simulink model "integrated"  (R2020b)
settings: Solver=VariableStepAuto  StartTime=0.0  StopTime=100  RelTol=1e-3
undefined symbols (not defined in the file or in its folder): sigbuilder_block
settings Model: EnablePacing=on  PacingRate=2  Creator=99003729  LastModifiedBy=99003729

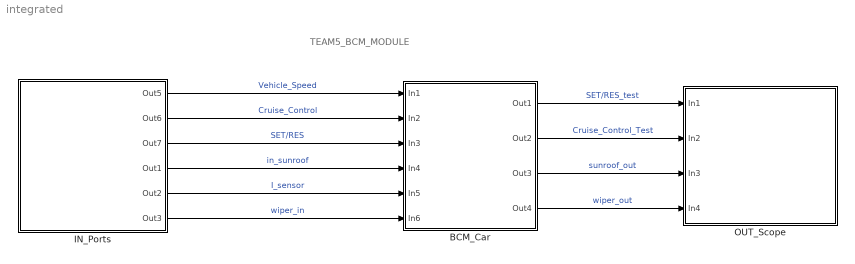
== system integrated ==
  note: TEAM5_BCM_MODULE
  BCM_Car : Subsystem
  IN_Ports : Subsystem
  OUT_Scope : Subsystem
  wires:
  IN_Ports/1(Out5) -> BCM_Car/1(In1)  "Vehicle_Speed"
  IN_Ports/3(Out7) -> BCM_Car/3(In3)  "SET/RES"
  IN_Ports/2(Out6) -> BCM_Car/2(In2)  "Cruise_Control"
  BCM_Car/1(Out1) -> OUT_Scope/1(In1)  "SET/RES_test"
  BCM_Car/2(Out2) -> OUT_Scope/2(In2)  "Cruise_Control_Test"
  IN_Ports/4(Out1) -> BCM_Car/4(In4)  "in_sunroof"
  IN_Ports/5(Out2) -> BCM_Car/5(In5)  "I_sensor"
  IN_Ports/6(Out3) -> BCM_Car/6(In6)  "wiper_in"
  BCM_Car/3(Out3) -> OUT_Scope/3(In3)  "sunroof_out"
  BCM_Car/4(Out4) -> OUT_Scope/4(In4)  "wiper_out"

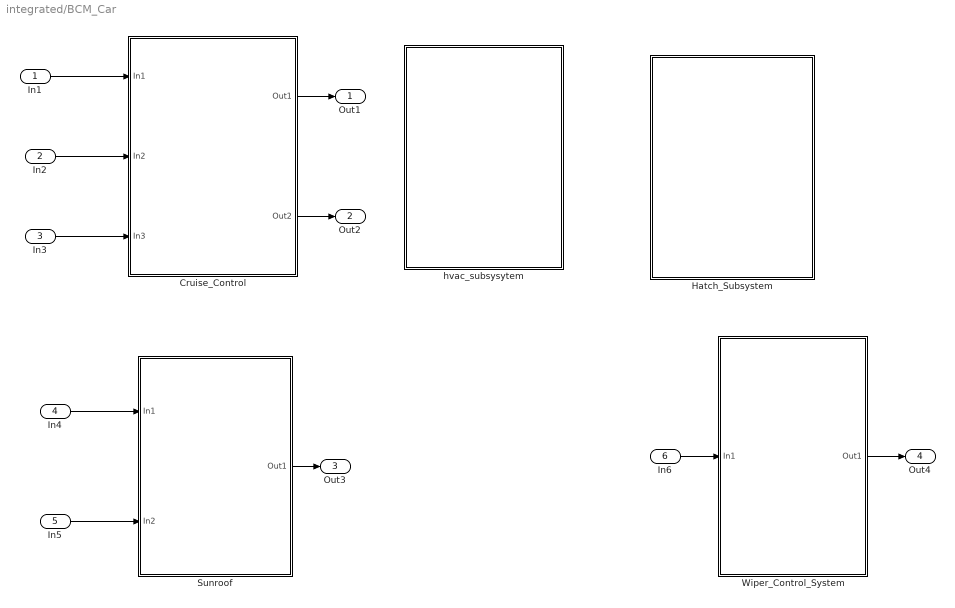
== system integrated/BCM_Car ==
  In1 : Inport
  In2 : Inport  Port=2
  In3 : Inport  Port=3
  In4 : Inport  Port=4
  In5 : Inport  Port=5
  In6 : Inport  Port=6
  Cruise_Control : Subsystem
  Hatch_Subsystem : Subsystem
  Sunroof : Subsystem
  Wiper_Control_System : Subsystem
  hvac_subsysytem : Subsystem
  Out1 : Outport
  Out2 : Outport  Port=2
  Out3 : Outport  Port=3
  Out4 : Outport  Port=4
  wires:
  In1/1 -> Cruise_Control/1(In1)
  In2/1 -> Cruise_Control/2(In2)
  In3/1 -> Cruise_Control/3(In3)
  Cruise_Control/1(Out1) -> Out1/1
  Cruise_Control/2(Out2) -> Out2/1
  In4/1 -> Sunroof/1(In1)
  In5/1 -> Sunroof/2(In2)
  Sunroof/1(Out1) -> Out3/1
  In6/1 -> Wiper_Control_System/1(In1)
  Wiper_Control_System/1(Out1) -> Out4/1

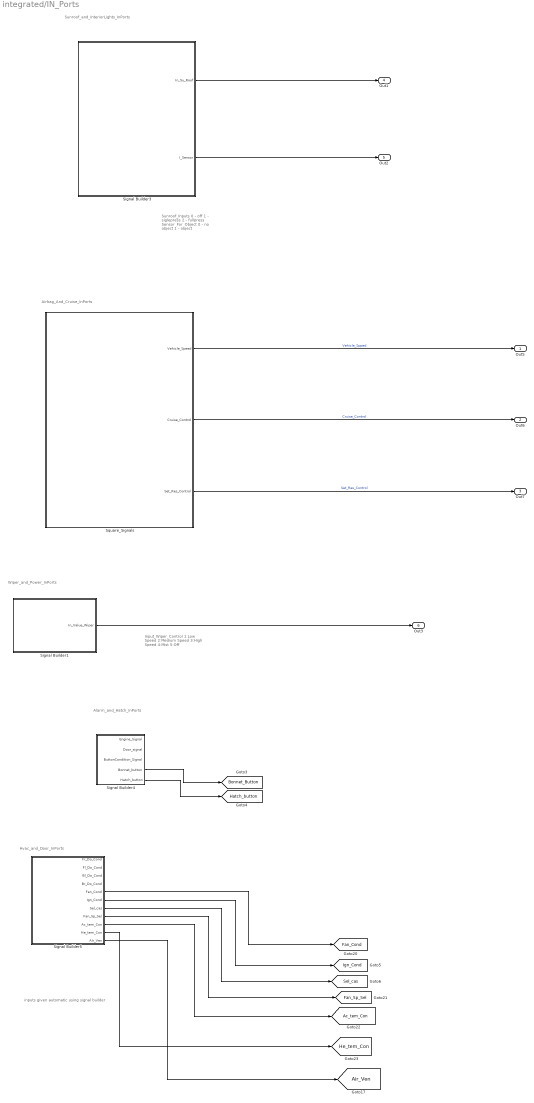
== system integrated/IN_Ports ==
  note: Hvac_and_Door_InPorts
  note: Alarm_and_Hatch_InPorts
  note: Sunroof_and_InteriorLights_InPorts
  note: Wiper_and_Power_InPorts
  note: Airbag_And_Cruise_InPorts
  note: Input_Wiper_Control
      | 1:Low Speed
      | 2:Medium Speed
      | 3:High Speed
      | 4:Mist
      | 5:Off
  note: Sunroof_Inputs
      | 0 - off
      | 1 - siglepress
      | 2 - fullpress
      | Sensor_For_Object
      | 0 - no object
      | 1 - object
  note: inputs given automatic using signal builder
  Signal Builder1 : Subsystem  Tag=STV Subsys  LoadFcn=sigbuilder_block('load');  StartFcn=sigbuilder_block('start');  StopFcn=sigbuilder_block('stop');  ClipboardFcn=sigbuilder_block('clipboard');  mask(Sigbuilder block){tuvar=[0:10]}
      mask help: Simulink:masks:SigbuilderBlock_MD
      mask init:
      | if ~strcmp(get_param(bdroot(gcbh),'SimulationStatus'),'stopped') tuvar = sigbuilder_block('maskInit'); end
      settings: CopyFcn=sigbuilder_block('copy');  DeleteFcn=sigbuilder_block('delete');  ModelCloseFcn=sigbuilder_block('modelClose');  PreSaveFcn=sigbuilder_block('preSave');  PauseFcn=sigbuilder_block('pause');  ContinueFcn=sigbuilder_block('continue');  NameChangeFcn=sigbuilder_block('namechange');  OpenFcn=sigbuilder_block('open',[0.75 30.75 718.5 715.5 ]);  CloseFcn=sigbuilder_block('close');
      mask Display: plot(0, 0, 100, 100,[2, 2, 32, 32, 2], [68, 8, 8, 68, 68],[32, 2], [38, 38], [32, 19, 2],[53, 60, 44], [32, 17, 17, 2],[16, 16, 31, 31]);txt = getActiveGroup(gcbh);text(2, 100, txt,'verticalAlignment', 'top');
  Signal Builder3 : Subsystem  Tag=STV Subsys  LoadFcn=sigbuilder_block('load');  StartFcn=sigbuilder_block('start');  StopFcn=sigbuilder_block('stop');  ClipboardFcn=sigbuilder_block('clipboard');  mask(Sigbuilder block){tuvar=[0:10]}
      mask help: Simulink:masks:SigbuilderBlock_MD
      mask init:
      | if ~strcmp(get_param(bdroot(gcbh),'SimulationStatus'),'stopped') tuvar = sigbuilder_block('maskInit'); end
      settings: CopyFcn=sigbuilder_block('copy');  DeleteFcn=sigbuilder_block('delete');  ModelCloseFcn=sigbuilder_block('modelClose');  PreSaveFcn=sigbuilder_block('preSave');  PauseFcn=sigbuilder_block('pause');  ContinueFcn=sigbuilder_block('continue');  NameChangeFcn=sigbuilder_block('namechange');  OpenFcn=sigbuilder_block('open',[591 352.5 550.5 359.25 ]);  CloseFcn=sigbuilder_block('close');
      mask Display: plot(0, 0, 100, 100,[2, 2, 32, 32, 2], [68, 8, 8, 68, 68],[32, 2], [38, 38], [32, 19, 2],[53, 60, 44], [32, 17, 17, 2],[16, 16, 31, 31]);txt = getActiveGroup(gcbh);text(2, 100, txt,'verticalAlignment', 'top');
  Signal Builder4 : Subsystem  Tag=STV Subsys  LoadFcn=sigbuilder_block('load');  StartFcn=sigbuilder_block('start');  StopFcn=sigbuilder_block('stop');  ClipboardFcn=sigbuilder_block('clipboard');  mask(Sigbuilder block){tuvar=[0:10]}
      mask help: Simulink:masks:SigbuilderBlock_MD
      mask init:
      | if ~strcmp(get_param(bdroot(gcbh),'SimulationStatus'),'stopped') tuvar = sigbuilder_block('maskInit'); end
      settings: CopyFcn=sigbuilder_block('copy');  DeleteFcn=sigbuilder_block('delete');  ModelCloseFcn=sigbuilder_block('modelClose');  PreSaveFcn=sigbuilder_block('preSave');  PauseFcn=sigbuilder_block('pause');  ContinueFcn=sigbuilder_block('continue');  NameChangeFcn=sigbuilder_block('namechange');  OpenFcn=sigbuilder_block('open',[437.6 199.2 550.4 400 ]);  CloseFcn=sigbuilder_block('close');
      mask Display: plot(0, 0, 100, 100,[2, 2, 32, 32, 2], [68, 8, 8, 68, 68],[32, 2], [38, 38], [32, 19, 2],[53, 60, 44], [32, 17, 17, 2],[16, 16, 31, 31]);txt = getActiveGroup(gcbh);text(2, 100, txt,'verticalAlignment', 'top');
  Signal Builder5 : Subsystem  Tag=STV Subsys  LoadFcn=sigbuilder_block('load');  StartFcn=sigbuilder_block('start');  StopFcn=sigbuilder_block('stop');  ClipboardFcn=sigbuilder_block('clipboard');  mask(Sigbuilder block){tuvar=[0:10]}
      mask help: Simulink:masks:SigbuilderBlock_MD
      mask init:
      | if ~strcmp(get_param(bdroot(gcbh),'SimulationStatus'),'stopped') tuvar = sigbuilder_block('maskInit'); end
      settings: CopyFcn=sigbuilder_block('copy');  DeleteFcn=sigbuilder_block('delete');  ModelCloseFcn=sigbuilder_block('modelClose');  PreSaveFcn=sigbuilder_block('preSave');  PauseFcn=sigbuilder_block('pause');  ContinueFcn=sigbuilder_block('continue');  NameChangeFcn=sigbuilder_block('namechange');  OpenFcn=sigbuilder_block('open',[544.5 115.5 550.5 399.75 ]);  CloseFcn=sigbuilder_block('close');
      mask Display: plot(0, 0, 100, 100,[2, 2, 32, 32, 2], [68, 8, 8, 68, 68],[32, 2], [38, 38], [32, 19, 2],[53, 60, 44], [32, 17, 17, 2],[16, 16, 31, 31]);txt = getActiveGroup(gcbh);text(2, 100, txt,'verticalAlignment', 'top');
  Square_Signals : Subsystem  Tag=STV Subsys  LoadFcn=sigbuilder_block('load');  StartFcn=sigbuilder_block('start');  StopFcn=sigbuilder_block('stop');  ClipboardFcn=sigbuilder_block('clipboard');  mask(Sigbuilder block){tuvar=[0:10]}
      mask help: Simulink:masks:SigbuilderBlock_MD
      mask init:
      | if ~strcmp(get_param(bdroot(gcbh),'SimulationStatus'),'stopped') tuvar = sigbuilder_block('maskInit'); end
      settings: CopyFcn=sigbuilder_block('copy');  DeleteFcn=sigbuilder_block('delete');  ModelCloseFcn=sigbuilder_block('modelClose');  PreSaveFcn=sigbuilder_block('preSave');  PauseFcn=sigbuilder_block('pause');  ContinueFcn=sigbuilder_block('continue');  NameChangeFcn=sigbuilder_block('namechange');  OpenFcn=sigbuilder_block('open',[6 30 1012.5 447.75 ]);  CloseFcn=sigbuilder_block('close');
      mask Display: plot(0, 0, 100, 100,[2, 2, 32, 32, 2], [68, 8, 8, 68, 68],[32, 2], [38, 38], [32, 19, 2],[53, 60, 44], [32, 17, 17, 2],[16, 16, 31, 31]);txt = getActiveGroup(gcbh);text(2, 100, txt,'verticalAlignment', 'top');
  Out5 : Outport
  Out6 : Outport  Port=2
  Out7 : Outport  Port=3
  Out1 : Outport  Port=4
  Out2 : Outport  Port=5
  Out3 : Outport  Port=6
  tag scope: Ac_tem_Con=global, Air_Ven=global, Bonnet_Button=global, Fan_Cond=global, Fan_Sp_Sel=global, Hatch_button=global, He_tem_Con=global, Ign_Cond=global, Sel_cas=global
  wires:
  Square_Signals/2(Cruise_Control) -> Out6/1  "Cruise_Control"
  Square_Signals/1(Vehicle_Speed) -> Out5/1  "Vehicle_Spped"
  Square_Signals/3(Set_Res_Control) -> Out7/1  "Set_Res_Control"
  Signal Builder1/1(In_Value_Wiper) -> Out3/1
  Signal Builder3/1(In_Su_Roof) -> Out1/1
  Signal Builder3/2(I_Sensor) -> Out2/1
  Signal Builder4/4(Bonnet_button) -> [Bonnet_Button]
  Signal Builder4/5(Hatch_button) -> [Hatch_button]
  Signal Builder5/10(He_tem_Con) -> [He_tem_Con]
  Signal Builder5/11(AIr_Ven) -> [Air_Ven]
  Signal Builder5/9(Ac_tem_Con) -> [Ac_tem_Con]
  Signal Builder5/5(Fan_Cond) -> [Fan_Cond]
  Signal Builder5/8(Fan_Sp_Sel) -> [Fan_Sp_Sel]
  Signal Builder5/7(Sel_cas) -> [Sel_cas]
  Signal Builder5/6(Ign_Cond) -> [Ign_Cond]

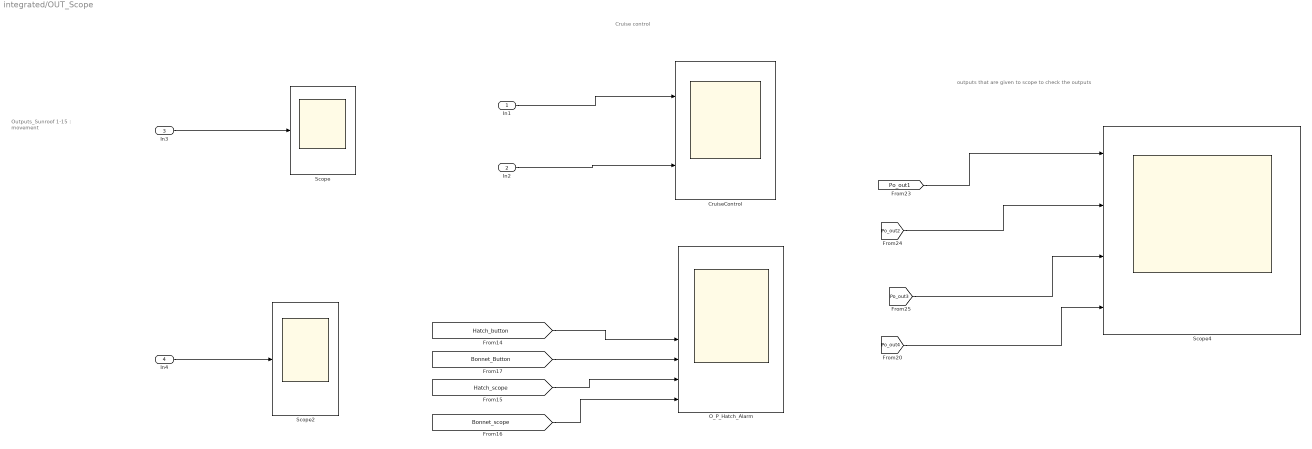
== system integrated/OUT_Scope ==
  note: Cruise control
  note: Outputs_Sunroof
      | 1-15 : movement
  note: outputs that are given to scope to check the outputs
  In1 : Inport
  In2 : Inport  Port=2
  In3 : Inport  Port=3
  In4 : Inport  Port=4
  CruiseControl : Scope  NumInputPorts=2
  O_P_Hatch_Alarm : Scope  NumInputPorts=8
  Scope : Scope
  Scope2 : Scope
  Scope4 : Scope  NumInputPorts=4
  wires:
  In4/1 -> Scope2/1
  In3/1 -> Scope/1
  [Bonnet_Button] -> O_P_Hatch_Alarm/6
  [Bonnet_scope] -> O_P_Hatch_Alarm/8
  [Hatch_button] -> O_P_Hatch_Alarm/5
  [Hatch_scope] -> O_P_Hatch_Alarm/7
  [Po_out3] -> Scope4/3
  [Po_out4] -> Scope4/4
  [Po_out1] -> Scope4/1
  [Po_out2] -> Scope4/2
  In1/1 -> CruiseControl/1
  In2/1 -> CruiseControl/2

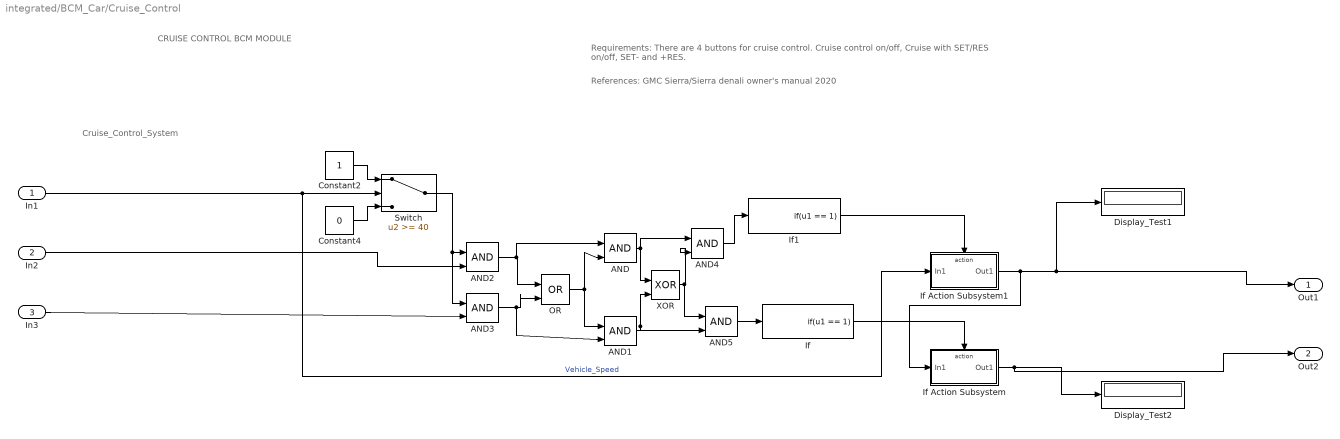
== system integrated/BCM_Car/Cruise_Control ==
  note: Cruise_Control_System
  note: CRUISE CONTROL BCM MODULE
  note: References: GMC Sierra/Sierra denali owner's manual 2020
  note: Requirements: There are 4 buttons for cruise control. Cruise control on/off, Cruise with SET/RES on/off, SET- and +RES.
  In1 : Inport
  In2 : Inport  Port=2
  In3 : Inport  Port=3
  AND{,1..5} (6 alike) : Logic  IconShape=distinctive  AllPortsSameDT=off  OutDataTypeStr=boolean
  Constant2 : Constant
  Constant4 : Constant  Value=0
  Display_Test1 : Display
  Display_Test2 : Display
  If : If  IfExpression=u1 == 1  ShowElse=off
  If Action Subsystem : Subsystem  TreatAsAtomicUnit=on
  If Action Subsystem1 : Subsystem  TreatAsAtomicUnit=on
  If1 : If  IfExpression=u1 == 1  ShowElse=off
  OR : Logic  Operator=OR  IconShape=distinctive  AllPortsSameDT=off  OutDataTypeStr=boolean
  Switch : Switch  Threshold=40
  XOR : Logic  Operator=XOR  IconShape=distinctive  AllPortsSameDT=off  OutDataTypeStr=boolean
  Out1 : Outport
  Out2 : Outport  Port=2
  wires:
  In3/1 -> AND3/2
  AND5/1 -> If/1
  If1/1 -> If Action Subsystem1/Action
  If/1 -> If Action Subsystem/Action
  If Action Subsystem/1(Out1) -> Out2/1, Display_Test2/1
  AND/1 -> AND4/1, XOR/1
  XOR/1 -> AND5/1, AND4/2
  In1/1 -> If Action Subsystem1/1(In1), Switch/2  "Vehicle_Speed"
  OR/1 -> AND1/1, AND/2
  AND2/1 -> AND/1, OR/1
  In2/1 -> AND2/2
  Constant4/1 -> Switch/3
  AND3/1 -> AND1/2, OR/2
  AND1/1 -> XOR/2, AND5/2
  Switch/1 -> AND3/1, AND2/1
  Constant2/1 -> Switch/1
  AND4/1 -> If1/1
  If Action Subsystem1/1(Out1) -> If Action Subsystem/1(In1), Out1/1, Display_Test1/1

== system integrated/BCM_Car/Hatch_Subsystem ==
  H_B_condition : Stateflow chart  TreatAsAtomicUnit=on
  Hatch_Bonnet_condition : Display
  OR : Logic  Operator=OR  IconShape=distinctive  AllPortsSameDT=off  OutDataTypeStr=boolean
  tag scope: Bonnet_scope=global, Hatch_scope=global
  wires:
  [Bonnet_Button] -> H_B_condition/1(BonnetButton)
  OR/1 -> Hatch_Bonnet_condition/1
  H_B_condition/1(y) -> [Bonnet_scope], OR/1
  H_B_condition/2(x) -> [Hatch_scope], OR/2
  [Hatch_button] -> H_B_condition/2(hatchButton)

== system integrated/BCM_Car/Sunroof ==
  In1 : Inport
  In2 : Inport  Port=2
  Function_Sun : MATLAB Function  TreatAsAtomicUnit=on
  Out1 : Outport
  wires:
  Function_Sun/1(y) -> Out1/1  "Out_Sun"
  In2/1 -> Function_Sun/2(v)
  In1/1 -> Function_Sun/1(u)

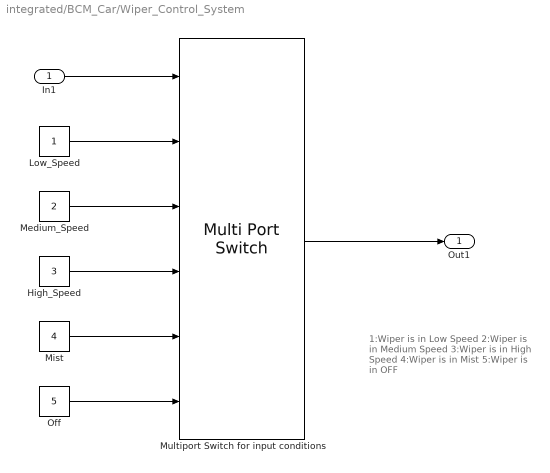
== system integrated/BCM_Car/Wiper_Control_System ==
  note: 1:Wiper is in Low Speed
      | 2:Wiper is in Medium Speed
      | 3:Wiper is in High Speed
      | 4:Wiper is in Mist
      | 5:Wiper is in OFF
  In1 : Inport
  High_Speed : Constant  Value=3
  Low_Speed : Constant
  Medium_Speed : Constant  Value=2
  Mist : Constant  Value=4
  Multiport Switch for input conditions : MultiPortSwitch  Inputs=5  DiagnosticForDefault=None
  Off : Constant  Value=5
  Out1 : Outport
  wires:
  In1/1 -> Multiport Switch for input conditions/1
  Low_Speed/1 -> Multiport Switch for input conditions/2
  Mist/1 -> Multiport Switch for input conditions/5
  Medium_Speed/1 -> Multiport Switch for input conditions/3
  Multiport Switch for input conditions/1 -> Out1/1
  High_Speed/1 -> Multiport Switch for input conditions/4
  Off/1 -> Multiport Switch for input conditions/6

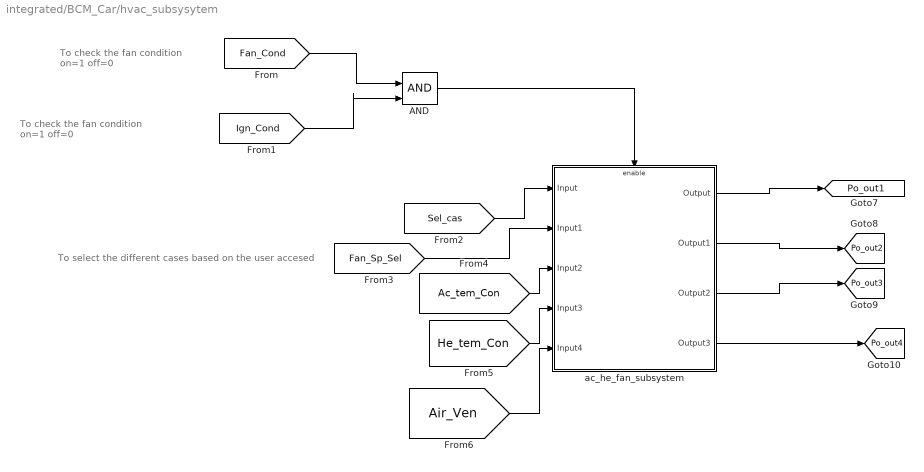
== system integrated/BCM_Car/hvac_subsysytem ==
  note: To select the different cases based on the user accesed
  note: To check the fan condition
      | on=1
      | off=0
  note: To check the fan condition
      | on=1
      | off=0
  AND : Logic  IconShape=distinctive  AllPortsSameDT=off  OutDataTypeStr=boolean
  ac_he_fan_subsystem : Subsystem
  tag scope: Po_out1=global, Po_out2=global, Po_out3=global, Po_out4=global
  wires:
  [Fan_Cond] -> AND/1
  [Ign_Cond] -> AND/2
  AND/1 -> ac_he_fan_subsystem/Enable
  [Sel_cas] -> ac_he_fan_subsystem/1(Input)
  [Fan_Sp_Sel] -> ac_he_fan_subsystem/2(Input1)
  [Ac_tem_Con] -> ac_he_fan_subsystem/3(Input2)
  [He_tem_Con] -> ac_he_fan_subsystem/4(Input3)
  ac_he_fan_subsystem/1(Output) -> [Po_out1]
  ac_he_fan_subsystem/2(Output1) -> [Po_out2]
  ac_he_fan_subsystem/3(Output2) -> [Po_out3]
  ac_he_fan_subsystem/4(Output3) -> [Po_out4]
  [Air_Ven] -> ac_he_fan_subsystem/5(Input4)

== system integrated/IN_Ports/Signal Builder1 ==
  Demux : Demux  Tag=STV Demux  Outputs=1
      settings: DisplayOption=none
  FromWs : FromWorkspace  Tag=STV FromWs  VariableName=tuvar
      SigBuilderData=|
      | common.afterFinalStr = 'Extrapolate'
      | common.sampleTime = 0
      | dataSet.timeRange = [0 25]
      | dataSet.name = 'Group 1'
      | sbobj.Groups.Name = 'Group 1'
      | sbobj.Groups.Signals.Name = 'In_Value_Wiper'
      | sbobj.Groups.Signals.XData = [0 1 2 3 4 5 6 7 8 9 10 11 12 13 14 15 16 17 18 19 20 21 22 23 24 25]
      | sbobj.Groups.Signals.YData = [1 4 3 4 5 3 1 2 1 4 1 2 5 3 2 3 5 1 4 3 5 1 2 4 3 5]
      | sbobj.Groups.TimeRange = [0 25]
  In_Value_Wiper : Outport  Tag=STV Outport
  wires:
  FromWs/1 -> Demux/1
  Demux/1 -> In_Value_Wiper/1

== system integrated/IN_Ports/Signal Builder3 ==
  Demux : Demux  Tag=STV Demux  Outputs=2
      settings: DisplayOption=none
  FromWs : FromWorkspace  Tag=STV FromWs  VariableName=tuvar
      SigBuilderData=|
      | common.afterFinalStr = 'Extrapolate'
      | common.sampleTime = 0
      | dataSet.timeRange = [0 10]
      | dataSet.name = 'Group 1'
      | sbobj.Groups.Name = 'Group 1'
      | sbobj.Groups.Signals(1).Name = 'In_Su_Roof'
      | sbobj.Groups.Signals(1).XData = [0 1 2 3 4 5 6 7 8 9 10]
      | sbobj.Groups.Signals(1).YData = [0 1 2 3 2 1 0 3 0 1 2]
      | sbobj.Groups.Signals(2).Name = 'I_Sensor'
      | sbobj.Groups.Signals(2).XData = [0 1 2 3 4 5 6 7 8 9 10]
      | sbobj.Groups.Signals(2).YData = [0 1 1 0 0 0 0 1 1 0 1]
  In_Su_Roof : Outport  Tag=STV Outport
  I_Sensor : Outport  Tag=STV Outport  Port=2
  wires:
  FromWs/1 -> Demux/1
  Demux/1 -> In_Su_Roof/1
  Demux/2 -> I_Sensor/1

== system integrated/IN_Ports/Signal Builder4 ==
  Demux : Demux  Tag=STV Demux  Outputs=5
      settings: DisplayOption=none
  FromWs : FromWorkspace  Tag=STV FromWs  VariableName=tuvar
      SigBuilderData=|
      | common.afterFinalStr = 'Extrapolate'
      | common.sampleTime = 0
      | dataSet.timeRange = [0 10]
      | dataSet.name = 'Group 1'
      | sbobj.Groups.Name = 'Group 1'
      | sbobj.Groups.Signals(1).Name = 'Engine_Signal'
      | sbobj.Groups.Signals(1).XData = [0 5 5 10 10 15 15 20 20 25 25 30 30 35 35 40 40 45 45 50 50 55 55 60 60 65 65 70 70 75 75 80 80 85 85 90 90 95 95 100]
      | sbobj.Groups.Signals(1).YData = [0 0 1 1 0 0 1 1 0 0 1 1 0 0 1 1 0 0 1 1 0 0 1 1 0 0 1 1 0 0 1 1 0 0 1 1 0 0 1 1]
      | sbobj.Groups.Signals(2).Name = 'Door_signal'
      | sbobj.Groups.Signals(2).XData = [0 5 5 10 10 15 15 20 20 25 25 30 30 35 35 40 40 45 45 50 50 55 55 60 60 65 65 70 70 75 75 80 80 85 85 90 90 95 95 100]
      | sbobj.Groups.Signals(2).YData = [1 1 0 0 1 1 0 0 1 1 0 0 1 1 0 0 1 1 0 0 1 1 0 0 1 1 0 0 1 1 0 0 1 1 0 0 1 1 0 0]
      | sbobj.Groups.Signals(3).Name = 'ButtonCondition_Signal'
      | sbobj.Groups.Signals(3).XData = [0 5 5 10 15 20 20 25 30 35 35 40 40 45 45 50 50 55 60 60 65 65 70 70 75 75 80 85 90 95 95 100]
      | sbobj.Groups.Signals(3).YData = [0 0 1 2 2 0 1 2 2 0 1 2 0 1 2 0 1 1 1 2 0 1 2 0 1 2 1 1 1 0 1 1]
      | sbobj.Groups.Signals(4).Name = 'Bonnet_button'
      | sbobj.Groups.Signals(4).XData = [0 5 5 10 10 15 15 20 20 25 25 30 30 35 35 40 40 45 45 50 50 55 55 60 60 65 65 70 70 75 75 80 80 85 85 90 90 95 95 100]
      | sbobj.Groups.Signals(4).YData = [0 0 1 1 0 0 1 1 0 0 1 1 0 0 1 1 0 0 1 1 0 0 1 1 0 0 1 1 0 0 1 1 0 0 1 1 0 0 1 1]
      | sbobj.Groups.Signals(5).Name = 'Hatch_button'
      | sbobj.Groups.Signals(5).XData = [0 5 5 10 10 15 15 20 20 25 25 30 30 35 35 40 40 45 45 50 50 55 55 60 60 65 65 70 70 75 75 80 80 85 85 90 90 95 95 100]
      | sbobj.Groups.Signals(5).YData = [1 1 0 0 1 1 0 0 1 1 0 0 1 1 0 0 1 1 0 0 1 1 0 0 1 1 0 0 1 1 0 0 1 1 0 0 1 1 0 0]
      | sbobj.Groups.TimeRange = [0 100]
  Engine_Signal : Outport  Tag=STV Outport
  Door_signal : Outport  Tag=STV Outport  Port=2
  ButtonCondition_Signal : Outport  Tag=STV Outport  Port=3
  Bonnet_button : Outport  Tag=STV Outport  Port=4
  Hatch_button : Outport  Tag=STV Outport  Port=5
  wires:
  FromWs/1 -> Demux/1
  Demux/1 -> Engine_Signal/1
  Demux/2 -> Door_signal/1
  Demux/3 -> ButtonCondition_Signal/1
  Demux/4 -> Bonnet_button/1
  Demux/5 -> Hatch_button/1

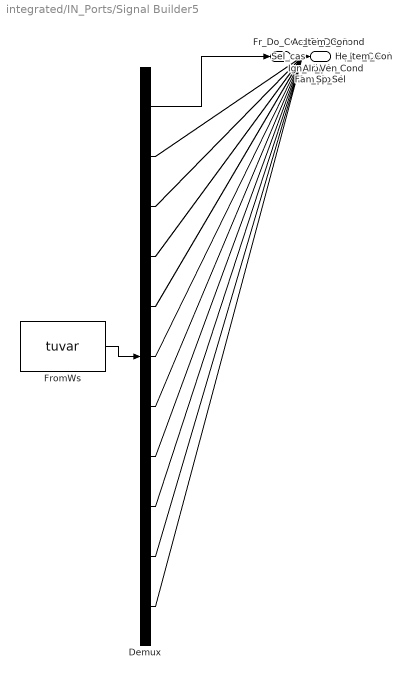
== system integrated/IN_Ports/Signal Builder5 ==
  Demux : Demux  Tag=STV Demux  Outputs=11
      settings: DisplayOption=none
  FromWs : FromWorkspace  Tag=STV FromWs  VariableName=tuvar
      SigBuilderData=|
      | common.afterFinalStr = 'Extrapolate'
      | common.sampleTime = 0
      | dataSet.timeRange = [0 10]
      | dataSet.name = 'Group 1'
      | sbobj.Groups.Name = 'Group 1'
      | sbobj.Groups.Signals(1).Name = 'Fr_Do_Cond'
      | sbobj.Groups.Signals(1).XData = [0 5 10 15 20 25 30 35 40]
      | sbobj.Groups.Signals(1).YData = [0 0 1 1 1 1 1 1 1]
      | sbobj.Groups.Signals(2).Name = 'Fl_Do_Cond'
      | sbobj.Groups.Signals(2).XData = [0 5 10 15 20 25 30 35 40]
      | sbobj.Groups.Signals(2).YData = [0 0 1 1 1 1 1 1 1]
      | sbobj.Groups.Signals(3).Name = 'Bl_Do_Cond'
      | sbobj.Groups.Signals(3).XData = [0 5 10 15 20 25 30 35 40]
      | sbobj.Groups.Signals(3).YData = [0 0 1 1 1 1 1 1 1]
      | sbobj.Groups.Signals(4).Name = 'Br_Do_Cond'
      | sbobj.Groups.Signals(4).XData = [0 5 10 15 20 25 30 35 40]
      | sbobj.Groups.Signals(4).YData = [0 0 1 1 1 1 1 1 1]
      | sbobj.Groups.Signals(5).Name = 'Fan_Cond'
      | sbobj.Groups.Signals(5).XData = [0 5 10 15 20 25 30 35 40]
      | sbobj.Groups.Signals(5).YData = [0 0 1 1 1 1 1 1 1]
      | sbobj.Groups.Signals(6).Name = 'Ign_Cond'
      | sbobj.Groups.Signals(6).XData = [0 5 10 15 20 25 30 35 40]
      | sbobj.Groups.Signals(6).YData = [0 0 1 1 1 1 1 1 1]
      | sbobj.Groups.Signals(7).Name = 'Sel_cas'
      | sbobj.Groups.Signals(7).XData = [0 5 10 15 20 25 30 35 40]
      | sbobj.Groups.Signals(7).YData = [1 1 2 3 1 2 3 1 2]
      | sbobj.Groups.Signals(8).Name = 'Fan_Sp_Sel'
      | sbobj.Groups.Signals(8).XData = [0 5 10 15 20 25 30 35 40]
      | sbobj.Groups.Signals(8).YData = [2 2 1 2 3 1 2 3 3]
      | sbobj.Groups.Signals(9).Name = 'Ac_tem_Con'
      | sbobj.Groups.Signals(9).XData = [0 5 10 15 20 25 30 35 40]
      | sbobj.Groups.Signals(9).YData = [25 25 32 25 28 30 20 18 16]
      | sbobj.Groups.Signals(10).Name = 'He_tem_Con'
      | sbobj.Groups.Signals(10).XData = [0 5 10 15 20 25 30 35 40]
      | sbobj.Groups.Signals(10).YData = [12 12 26 35 34 32 35 31 32]
      | sbobj.Groups.Signals(11).Name = 'AIr_Ven'
      | sbobj.Groups.Signals(11).XData = [0 5 10 15 20 25 30 35 40]
      | sbobj.Groups.Signals(11).YData = [50 50 100 50 0 100 0 50 100]
      | sbobj.Groups.TimeRange = [0 40]
  Fr_Do_Cond : Outport  Tag=STV Outport
  Fl_Do_Cond : Outport  Tag=STV Outport  Port=2
  Bl_Do_Cond : Outport  Tag=STV Outport  Port=3
  Br_Do_Cond : Outport  Tag=STV Outport  Port=4
  Fan_Cond : Outport  Tag=STV Outport  Port=5
  Ign_Cond : Outport  Tag=STV Outport  Port=6
  Sel_cas : Outport  Tag=STV Outport  Port=7
  Fan_Sp_Sel : Outport  Tag=STV Outport  Port=8
  Ac_tem_Con : Outport  Tag=STV Outport  Port=9
  He_tem_Con : Outport  Tag=STV Outport  Port=10
  AIr_Ven : Outport  Tag=STV Outport  Port=11
  wires:
  FromWs/1 -> Demux/1
  Demux/1 -> Fr_Do_Cond/1
  Demux/2 -> Fl_Do_Cond/1
  Demux/3 -> Bl_Do_Cond/1
  Demux/4 -> Br_Do_Cond/1
  Demux/5 -> Fan_Cond/1
  Demux/6 -> Ign_Cond/1
  Demux/7 -> Sel_cas/1
  Demux/8 -> Fan_Sp_Sel/1
  Demux/9 -> Ac_tem_Con/1
  Demux/10 -> He_tem_Con/1
  Demux/11 -> AIr_Ven/1

== system integrated/IN_Ports/Square_Signals ==
  Demux : Demux  Tag=STV Demux  Outputs=3
      settings: DisplayOption=none
  FromWs : FromWorkspace  Tag=STV FromWs  VariableName=tuvar
      SigBuilderData=|
      | common.afterFinalStr = 'Extrapolate'
      | common.sampleTime = 0
      | dataSet.timeRange = [0 100]
      | dataSet.name = 'Group 1'
      | sbobj.Groups.Name = 'Group 1'
      | sbobj.Groups.Signals(1).Name = 'Vehicle_Speed'
      | sbobj.Groups.Signals(1).XData = [0 5 10 15 20 25 30 35 40 45 50 55 60 65 70 75 80 85 90 95 100]
      | sbobj.Groups.Signals(1).YData = [50 50 50 50 50 50 50 50 50 50 50 50 50 50 50 50 50 50 50 50 50]
      | sbobj.Groups.Signals(2).Name = 'Cruise_Control'
      | sbobj.Groups.Signals(2).XData = [0 5 5 10 15 20 25 30 35 40 45 50 55 60 65 70 75 80 85 90 95 100]
      | sbobj.Groups.Signals(2).YData = [0 0 1 1 1 1 1 0 0 0 0 0 0 0 0 0 0 0 0 0 0 0]
      | sbobj.Groups.Signals(3).Name = 'Set_Res_Control'
      | sbobj.Groups.Signals(3).XData = [0 5 10 15 20 25 30 30 35 35 40 45 50 55 60 65 70 75 80 85 90 95 100]
      | sbobj.Groups.Signals(3).YData = [0 0 0 0 0 0 0 1 1 0 0 0 0 0 0 0 0 0 0 0 0 0 0]
      | sbobj.Groups.TimeRange = [0 100]
  Vehicle_Speed : Outport  Tag=STV Outport
  Cruise_Control : Outport  Tag=STV Outport  Port=2
  Set_Res_Control : Outport  Tag=STV Outport  Port=3
  wires:
  FromWs/1 -> Demux/1
  Demux/1 -> Vehicle_Speed/1
  Demux/2 -> Cruise_Control/1
  Demux/3 -> Set_Res_Control/1

== system integrated/BCM_Car/Cruise_Control/If Action Subsystem ==
  In1 : Inport
  Action Port : ActionPort  ActionPortLabel=if(u1 == 1)
  Out1 : Outport
  wires:
  In1/1 -> Out1/1

== system integrated/BCM_Car/Cruise_Control/If Action Subsystem1 ==
  In1 : Inport
  Action Port : ActionPort  ActionPortLabel=if(u1 == 1)
  Add : Sum
  Chart : Stateflow chart  TreatAsAtomicUnit=on
  Signal Builder : Subsystem  Tag=STV Subsys  LoadFcn=sigbuilder_block('load');  StartFcn=sigbuilder_block('start');  StopFcn=sigbuilder_block('stop');  ClipboardFcn=sigbuilder_block('clipboard');  mask(Sigbuilder block){tuvar=[0:10]}
      mask help: Simulink:masks:SigbuilderBlock_MD
      mask init:
      | if ~strcmp(get_param(bdroot(gcbh),'SimulationStatus'),'stopped') tuvar = sigbuilder_block('maskInit'); end
      settings: CopyFcn=sigbuilder_block('copy');  DeleteFcn=sigbuilder_block('delete');  ModelCloseFcn=sigbuilder_block('modelClose');  PreSaveFcn=sigbuilder_block('preSave');  PauseFcn=sigbuilder_block('pause');  ContinueFcn=sigbuilder_block('continue');  NameChangeFcn=sigbuilder_block('namechange');  OpenFcn=sigbuilder_block('open',[0.75 30.75 718.5 715.5 ]);  CloseFcn=sigbuilder_block('close');
      mask Display: plot(0, 0, 100, 100,[2, 2, 32, 32, 2], [68, 8, 8, 68, 68],[32, 2], [38, 38], [32, 19, 2],[53, 60, 44], [32, 17, 17, 2],[16, 16, 31, 31]);txt = getActiveGroup(gcbh);text(2, 100, txt,'verticalAlignment', 'top');
  Out1 : Outport
  wires:
  Signal Builder/1(Plus_Or_Resume) -> Chart/2(inc)
  Add/1 -> Out1/1
  Signal Builder/2(Set_Or_Minus) -> Chart/1(dec)
  Chart/1(data) -> Add/1
  In1/1 -> Add/2

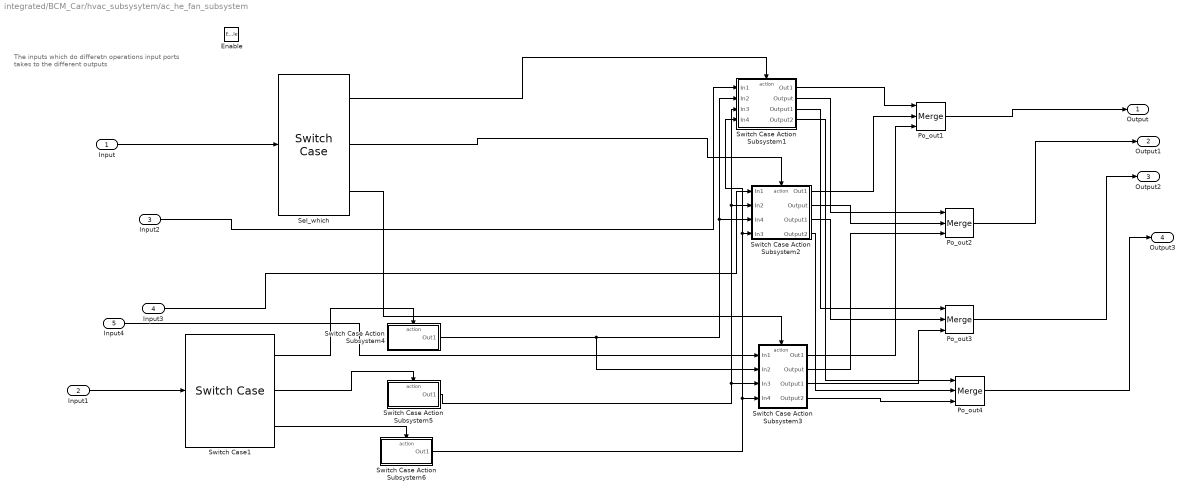
== system integrated/BCM_Car/hvac_subsysytem/ac_he_fan_subsystem ==
  note: The inputs which do differetn operations
      | input ports takes to the different outputs
  Input : Inport
  Input1 : Inport  Port=2
  Input2 : Inport  Port=3
  Input3 : Inport  Port=4
  Input4 : Inport  Port=5
  Enable : EnablePort
  Po_out{1..4} (4 alike) : Merge  Inputs=3
  "Sel_which " : SwitchCase  CaseConditions={1,2,3}  ShowDefaultCase=off
  Switch Case Action Subsystem1 : Subsystem  TreatAsAtomicUnit=on
  Switch Case Action Subsystem2 : Subsystem  TreatAsAtomicUnit=on
  Switch Case Action Subsystem3 : Subsystem  TreatAsAtomicUnit=on
  Switch Case Action Subsystem4 : Subsystem  TreatAsAtomicUnit=on
  Switch Case Action Subsystem5 : Subsystem  TreatAsAtomicUnit=on
  Switch Case Action Subsystem6 : Subsystem  TreatAsAtomicUnit=on
  Switch Case1 : SwitchCase  CaseConditions={1,2,3}  ShowDefaultCase=off
  Output : Outport
  Output1 : Outport  Port=2
  Output2 : Outport  Port=3
  Output3 : Outport  Port=4
  wires:
  Input/1 -> "Sel_which "/1
  Input2/1 -> Switch Case Action Subsystem1/1(In1)
  Input3/1 -> Switch Case Action Subsystem2/1(In1)
  Input4/1 -> Switch Case Action Subsystem3/1(In1)
  Input1/1 -> Switch Case1/1
  Switch Case1/2 -> Switch Case Action Subsystem5/Action
  Switch Case1/1 -> Switch Case Action Subsystem4/Action
  Switch Case1/3 -> Switch Case Action Subsystem6/Action
  Switch Case Action Subsystem4/1(Out1) -> Switch Case Action Subsystem3/2(In2), Switch Case Action Subsystem1/2(In2), Switch Case Action Subsystem2/3(In4)
  Switch Case Action Subsystem5/1(Out1) -> Switch Case Action Subsystem1/3(In3), Switch Case Action Subsystem2/2(In2), Switch Case Action Subsystem3/3(In3)
  Switch Case Action Subsystem6/1(Out1) -> Switch Case Action Subsystem3/4(In4), Switch Case Action Subsystem1/4(In4), Switch Case Action Subsystem2/4(In3)
  "Sel_which "/1 -> Switch Case Action Subsystem1/Action
  "Sel_which "/2 -> Switch Case Action Subsystem2/Action
  "Sel_which "/3 -> Switch Case Action Subsystem3/Action
  Switch Case Action Subsystem1/1(Out1) -> Po_out1/1
  Switch Case Action Subsystem2/1(Out1) -> Po_out1/2
  Switch Case Action Subsystem3/1(Out1) -> Po_out1/3
  Switch Case Action Subsystem1/2(Output) -> Po_out2/1
  Switch Case Action Subsystem2/2(Output) -> Po_out2/2
  Switch Case Action Subsystem3/2(Output) -> Po_out2/3
  Switch Case Action Subsystem1/3(Output1) -> Po_out3/1
  Switch Case Action Subsystem2/3(Output1) -> Po_out3/2
  Switch Case Action Subsystem3/3(Output1) -> Po_out3/3
  Switch Case Action Subsystem1/4(Output2) -> Po_out4/1
  Switch Case Action Subsystem2/4(Output2) -> Po_out4/2
  Switch Case Action Subsystem3/4(Output2) -> Po_out4/3
  Po_out1/1 -> Output/1
  Po_out2/1 -> Output1/1
  Po_out3/1 -> Output2/1
  Po_out4/1 -> Output3/1

== system integrated/BCM_Car/Cruise_Control/If Action Subsystem1/Signal Builder ==
  Demux : Demux  Tag=STV Demux  Outputs=2
      settings: DisplayOption=none
  FromWs : FromWorkspace  Tag=STV FromWs  VariableName=tuvar
      SigBuilderData=|
      | common.afterFinalStr = 'Extrapolate'
      | common.sampleTime = 0
      | dataSet.timeRange = [0 10]
      | dataSet.name = 'Group 1'
      | sbobj.Groups.Name = 'Group 1'
      | sbobj.Groups.Signals(1).Name = 'Plus_Or_Resume'
      | sbobj.Groups.Signals(1).XData = [0 5 5 10 15 20 20 25 30 30 35 35 40 45 50 55 60 65 70 75 80 85 90 95 100]
      | sbobj.Groups.Signals(1).YData = [0 0 1 1 1 1 0 0 0 1 1 0 0 0 0 0 0 0 0 0 0 0 0 0 0]
      | sbobj.Groups.Signals(2).Name = 'Set_Or_Minus'
      | sbobj.Groups.Signals(2).XData = [0 5 10 15 20 20 25 30 30 35 35 40 45 50 55 60 65 70 75 80 85 90 95 100]
      | sbobj.Groups.Signals(2).YData = [0 0 0 0 0 1 1 0 1 1 0 0 0 0 0 0 0 0 0 0 0 0 0 0]
      | sbobj.Groups.TimeRange = [0 100]
  Plus_Or_Resume : Outport  Tag=STV Outport
  Set_Or_Minus : Outport  Tag=STV Outport  Port=2
  wires:
  FromWs/1 -> Demux/1
  Demux/1 -> Plus_Or_Resume/1
  Demux/2 -> Set_Or_Minus/1

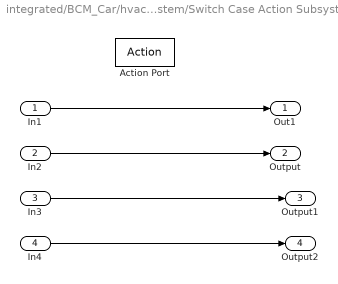
== system integrated/BCM_Car/hvac_subsysytem/ac_he_fan_subsystem/Switch Case Action Subsystem1 ==
  In1 : Inport
  In2 : Inport  Port=2
  In3 : Inport  Port=3
  In4 : Inport  Port=4
  Action Port : ActionPort  ActionPortLabel=case [ 1 ]:
  Out1 : Outport
  Output : Outport  Port=2
  Output1 : Outport  Port=3
  Output2 : Outport  Port=4
  wires:
  In1/1 -> Out1/1
  In2/1 -> Output/1
  In3/1 -> Output1/1
  In4/1 -> Output2/1

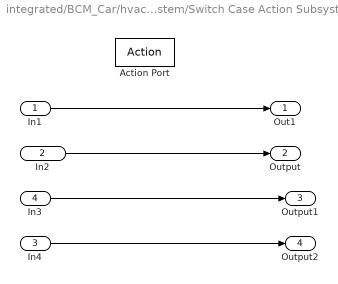
== system integrated/BCM_Car/hvac_subsysytem/ac_he_fan_subsystem/Switch Case Action Subsystem2 ==
  In1 : Inport
  In2 : Inport  Port=2
  In4 : Inport  Port=3
  In3 : Inport  Port=4
  Action Port : ActionPort  ActionPortLabel=case [ 2 ]:
  Out1 : Outport
  Output : Outport  Port=2
  Output1 : Outport  Port=3
  Output2 : Outport  Port=4
  wires:
  In1/1 -> Out1/1
  In2/1 -> Output/1
  In3/1 -> Output1/1
  In4/1 -> Output2/1

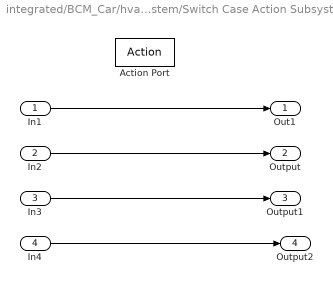
== system integrated/BCM_Car/hvac_subsysytem/ac_he_fan_subsystem/Switch Case Action Subsystem3 ==
  In1 : Inport
  In2 : Inport  Port=2
  In3 : Inport  Port=3
  In4 : Inport  Port=4
  Action Port : ActionPort  ActionPortLabel=case [ 3 ]:
  Out1 : Outport
  Output : Outport  Port=2
  Output1 : Outport  Port=3
  Output2 : Outport  Port=4
  wires:
  In1/1 -> Out1/1
  In2/1 -> Output/1
  In3/1 -> Output1/1
  In4/1 -> Output2/1

== system integrated/BCM_Car/hvac_subsysytem/ac_he_fan_subsystem/Switch Case Action Subsystem4 ==
  Action Port : ActionPort  ActionPortLabel=case [ 1 ]:
  Constant : Constant
  Out1 : Outport
  wires:
  Constant/1 -> Out1/1

== system integrated/BCM_Car/hvac_subsysytem/ac_he_fan_subsystem/Switch Case Action Subsystem5 ==
  Action Port : ActionPort  ActionPortLabel=case [ 2 ]:
  Constant : Constant
  Out1 : Outport
  wires:
  Constant/1 -> Out1/1

== system integrated/BCM_Car/hvac_subsysytem/ac_he_fan_subsystem/Switch Case Action Subsystem6 ==
  Action Port : ActionPort  ActionPortLabel=case [ 3 ]:
  Constant : Constant
  Out1 : Outport
  wires:
  Constant/1 -> Out1/1

== stateflow chart integrated/BCM_Car/Cruise_Control/If Action Subsystem1/Chart ==
  state main
    during:
    if inc==1
    data=data+1;
    end
    if dec==1
    data=data-1;
    end
  (default) -> main
  data: dec input; inc input; data output =0

== matlab function integrated/BCM_Car/Sunroof/Function_Sun ==
  data: u input; y output; v input
function y = fcn(u,v)
if u == 1
    for i = 1:5
        y = u * i;
    end
elseif u == 2
    for i = 1:5
        y = u * i;
    end
elseif u == 3
    for i = 1:5
        y = u * i;
    end
else
    y = u;
end
if v == 1 && u ~= 0
   y = 15;
end

== stateflow chart integrated/BCM_Car/Hatch_Subsystem/H_B_condition ==
  state Hatch
    entry:
    if hatchButton==1
    y=1;
    end
    if BonnetButton==1
    x=1;
    end
  state Hatch_off
    entry:
    if hatchButton==0
    y=0;
    end
    if BonnetButton==0
    x=0;
    end
  (default) -> Hatch
  Hatch -> Hatch_off : [BonnetButton==0||hatchButton==0]
  Hatch_off -> Hatch : [BonnetButton==1||hatchButton==1]
  data: BonnetButton input; hatchButton input; y output; x output
